simulink model "my_pv_system_3_ss_controller"  (Simulink 8.4)
settings: Solver=ode3  StartTime=0.0  StopTime=inf  FixedStep=5e-05  RelTol=1e-3
undefined symbols (not defined in the file or in its folder): another_event_name, my_event_name
libraries: powerlib_meascontrol x7, opal_lib x6, simulink x2, rtlab x1, powerlib x1
Description:
  | Model of a simple control system for use iin training.
settings Model: Creator=Paul Baracos  LastModifiedBy=jiang  BufferReuse=off
settings DataIOCC: SaveOutput=off  SaveTime=off  SignalLoggingName=sigsOut
settings OptimizationCC: BlockReduction=off  BooleanDataType=off  OptimizeBlockIOStorage=off  BufferReuse=off  GlobalBufferReuse=off  ExpressionFolding=off  ExpressionDepthLimit=128  LocalBlockOutputs=off  InitFltsAndDblsToZero=on
settings DebuggingCC: SaveWithParameterizedLinksMsg=none  SignalResolutionControl=TryResolveAllWithWarning  SolverPrmCheckMsg=none  MultiTaskDSMMsg=warning  MultiTaskCondExecSysMsg=none  StateNameClashWarn=none
settings HardwareCC: TargetHWDeviceType=32-bit Generic  TargetUnknown=on  ProdEqTarget=off
settings RTWCC: GenCodeOnly=on  IncludeERTFirstTime=on
settings GRTTargetCC: TargetFcnLib=ansi_tfl_tmw.mat
settings ConfigurationSet: Description=SimMechanics 2G

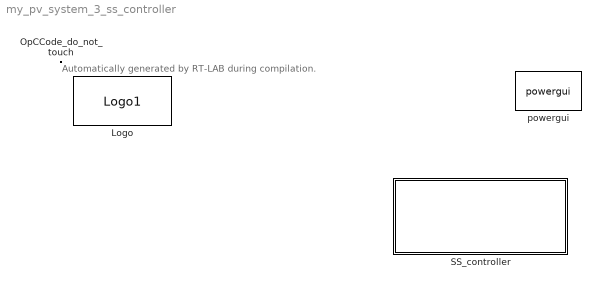
== system my_pv_system_3_ss_controller ==
  note: Automatically generated by RT-LAB during compilation.
  Logo : opal_lib/Logo1  vide=[]
  OpCCode_do_not_touch : opal_lib/Communication/OpCCode  SystemSampleTime=-1
  SS_controller : Subsystem
  powergui : powerlib/powergui  SimulationMode=Discrete  SolverType=Tustin/Backward Euler (TBE)  SampleTime=5e-05  frequency=60  SPID=off  DisableSnubberDevices=off  DisableRonSwitches=off  DisableVfSwitches=off  SwTol=0  DisplayEquations=off  Interpol=off  methode=off  Ts=100  frequencyindice=50  Pbase=100e6  ErrMax=1e-4  Iterations=50  UnitsV=kV  UnitsW=MW  FunctionMessages=off  echomessages=off  HookPort=off  EnableUseOfTLC=off  x0status=blocks  RestoreLinks=warning  ResistiveCurrentMeasurement=off  Frange=[0:2:500]  Ylog=off  Xlog=on  ShowGrid=off  save=off  variable=ZData  structure=0  ZoomFFT=off  StartTime=0.0  cycles=1  DisplayStyle=1  fundamental=60  FreqAxis=off  MaxFrequency=1000  frequencyindicesteady=1  RmsSteady=1  display=off

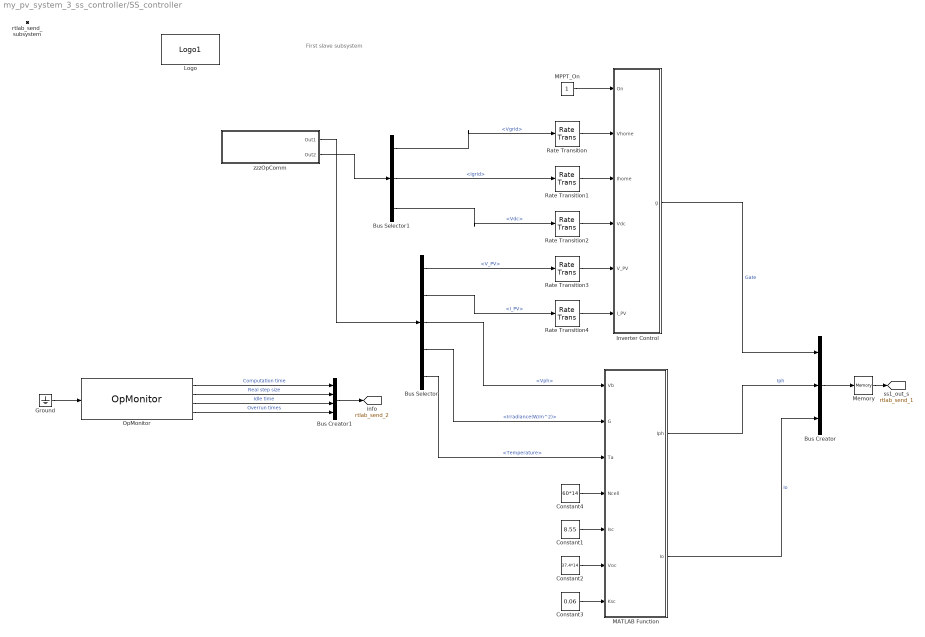
== system my_pv_system_3_ss_controller/SS_controller ==
  note: First slave subsystem
  Bus Creator : BusCreator  Inputs=3
  Bus Creator1 : BusCreator
  Bus Selector : BusSelector  OutputSignals=V_PV,I_PV,Vph,Irradiance(W/m^2),Temperature
  Bus Selector1 : BusSelector  OutputSignals=Vgrid,Igrid,Vdc
  Constant1 : Constant  Value=8.55
  Constant2 : Constant  Value=37.4*14
  Constant3 : Constant  Value=0.06
  Constant4 : Constant  Value=60*14
  Ground : Ground
  Inverter Control : Subsystem  mask(Inverter Control){Pnom=3500, Fnom=50, Vnom_prim=240, Vnom_dc=400, Increment_MPPT=0.003, Limits_MPPT=[ 450 375 ], Vdc_ref_Init=425, Kp_VDCreg=12, Ki_VDCreg=200, Kp_Ireg=0.15, Ki_Ireg=6.6, RLff=[ 0.002 0.20 ], Fc=4000, PWMmode12=Unipolar, Ts_Control=50e-6, Ts_PWMgenerator=50e-6}
      mask prompts: Pnom "Power (VA)"; Fnom "Frequency (Hz)"; Vnom_prim "Primary voltage (Vrms LL)"; Vnom_dc "DC voltage (V)"; Increment_MPPT "Output increment (V)"; Limits_MPPT "Output limits [ Upper  Lower ]"; Vdc_ref_Init "Output initial value (V)"; Kp_VDCreg "Proportional gain"; Ki_VDCreg "Integral gain"; Kp_Ireg "Proportional gain"; Ki_Ireg "Integral gain"; RLff "Feedforward Values [Rff Lff] (pu)"; Fc "Carrier frequency (Hz)"; PWMmode12 "PWM method"; Ts_Control "Control systems"; Ts_PWMgenerator "PWM generator"
      mask help:
      | The main components of the Inverter Control are:
      | 1. PLL & Measurements
      | 2. Maximum Power Point Tracker System (MPPT) using a Perturb & Observe algorithm
      | 3. DC Voltage Regulator
      | 4. Current Regulator
      | 5. PWM Modulator
      mask init:
      | blockName=gcb;
      | if PWMmode12==1
      |     set_param([blockName,'/','PWM_Generator'],'ModulatorType','Single-phase full-bridge (4 pulses)')
      | else
      |     set_param([blockName,'/','PWM_Generator'],'ModulatorType','Single-phase full-bridge - Bipolar modulation (4 pulses)')
      | end
      mask TypeOptions PWMmode12: Unipolar | Bipolar
  Logo : opal_lib/Logo1  vide=[]
  MATLAB Function : MATLAB Function  TreatAsAtomicUnit=on
  MPPT_On : Constant
  Memory : Memory  InheritSampleTime=on
  OpMonitor : rtlab/Monitoring/OpMonitor  compute_time=on  real_step=on  idle_time=on  nb_overruns=on  user_time=off  user_name=my_event_name,another_event_name
  Rate Transition{,1..4} (5 alike) : RateTransition
  rtlab_send_subsystem : Subsystem  Priority=-100
      mask Display: text(0,0,'');
  zzzOpComm : Subsystem
      mask init:
      | opmaskdisplay('maskdisplay_block',gcb,'disp(''OpComm'')');
      mask Display:
      | patch([0 0.5 0.7 0],[1 1 0 0],[0.7 0.75 0.9]);
      | patch([1 0.53 0.73 1],[1 1 0 0],[1 0.8 0.7]);
      | plot([0 0 1 1 0],[0 1 1 0 0]);
      | disp('OpComm')
  tag scope: rtlab_send_1=global, rtlab_send_2=global
  wires:
  Memory/1 -> [rtlab_send_1]
  MPPT_On/1 -> Inverter Control/1(On)
  Rate Transition/1 -> Inverter Control/2(Vhome)
  Rate Transition1/1 -> Inverter Control/3(Ihome)
  Rate Transition2/1 -> Inverter Control/4(Vdc)
  Rate Transition3/1 -> Inverter Control/5(V_PV)
  Rate Transition4/1 -> Inverter Control/6(I_PV)
  zzzOpComm/2(Out2) -> Bus Selector1/1
  Bus Selector1/1 -> Rate Transition/1  "<Vgrid>"
  Bus Selector1/2 -> Rate Transition1/1  "<Igrid>"
  Bus Selector1/3 -> Rate Transition2/1  "<Vdc>"
  zzzOpComm/1(Out1) -> Bus Selector/1
  Bus Selector/1 -> Rate Transition3/1  "<V_PV>"
  Bus Selector/2 -> Rate Transition4/1  "<I_PV>"
  Constant4/1 -> MATLAB Function/4(Ncell)
  Constant1/1 -> MATLAB Function/5(Isc)
  Constant2/1 -> MATLAB Function/6(Voc)
  Constant3/1 -> MATLAB Function/7(Ksc)
  Bus Creator/1 -> Memory/1
  Inverter Control/1(g) -> Bus Creator/1  "Gate"
  MATLAB Function/1(Iph) -> Bus Creator/2  "Iph"
  MATLAB Function/2(Io) -> Bus Creator/3  "Io"
  Bus Selector/3 -> MATLAB Function/1(Vb)  "<Vph>"
  Bus Selector/4 -> MATLAB Function/2(G)  "<Irradiance(W/m^2)>"
  Bus Selector/5 -> MATLAB Function/3(Ta)  "<Temperature>"
  Bus Creator1/1 -> [rtlab_send_2]
  OpMonitor/3 -> Bus Creator1/3  "Idle time"
  OpMonitor/1 -> Bus Creator1/1  "Computation time"
  OpMonitor/2 -> Bus Creator1/2  "Real step size"
  OpMonitor/4 -> Bus Creator1/4  "Overrun times"
  Ground/1 -> OpMonitor/1

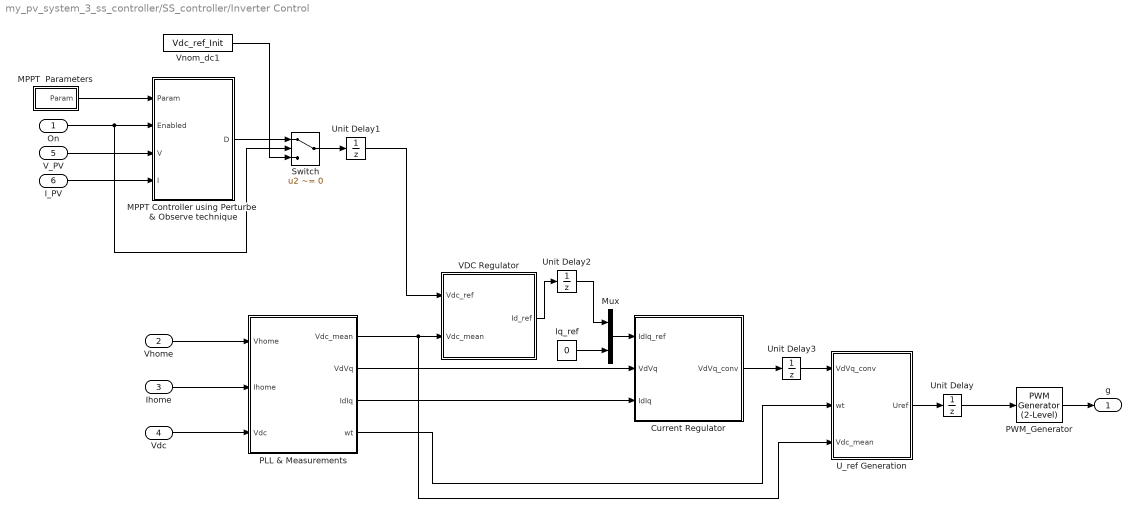
== system my_pv_system_3_ss_controller/SS_controller/Inverter Control ==
  On : Inport  PortDimensions=1
  Vhome : Inport  Port=2  PortDimensions=1
  Ihome : Inport  Port=3  PortDimensions=1
  Vdc : Inport  Port=4  PortDimensions=1
  V_PV : Inport  Port=5  PortDimensions=1
  I_PV : Inport  Port=6  PortDimensions=1
  Current Regulator : Subsystem
  Iq_ref : Constant  Value=0
  MPPT  Parameters : Subsystem
  "MPPT Controller using Perturbe  & Observe technique  " : MATLAB Function  TreatAsAtomicUnit=on
  Mux : Mux  Inputs=2
  PLL & Measurements : Subsystem
  PWM_Generator : powerlib_meascontrol/Pulse & Signal Generators/PWM Generator (2-Level)  ModulatorType=Single-phase full-bridge (4 pulses)  ModulatorMode=Unsynchronized  Fc=Fc  Pc=90  nF=27  MinMax="[ -1  1 ]"  SamplingTechnique=Natural  ModulatingSignals=off  m=0.8  Freq=60  Phase=0  Ts=Ts_PWMgenerator  ShowCarrierOutport=off
      settings: AttributesFormatString=%<ModulatorType>
  Switch : Switch  Criteria=u2 ~= 0
  "U_ref Generation " : Subsystem
  Unit Delay : UnitDelay  InitialCondition=0.1684  SampleTime=Ts_Control
  Unit Delay1 : UnitDelay  SampleTime=Ts_Control
  Unit Delay2 : UnitDelay  SampleTime=Ts_Control
  Unit Delay3 : UnitDelay  SampleTime=Ts_Control
  VDC Regulator : Subsystem
  Vnom_dc1 : Constant  Value=Vdc_ref_Init
  g : Outport
  wires:
  Iq_ref/1 -> Mux/2
  Vhome/1 -> PLL & Measurements/1(Vhome)
  Ihome/1 -> PLL & Measurements/2(Ihome)
  V_PV/1 -> "MPPT Controller using Perturbe  & Observe technique  "/3(V)
  I_PV/1 -> "MPPT Controller using Perturbe  & Observe technique  "/4(I)
  MPPT  Parameters/1(Param) -> "MPPT Controller using Perturbe  & Observe technique  "/1(Param)
  On/1 -> "MPPT Controller using Perturbe  & Observe technique  "/2(Enabled), Switch/2
  Unit Delay/1 -> PWM_Generator/1
  "MPPT Controller using Perturbe  & Observe technique  "/1(D) -> Switch/1
  Vdc/1 -> PLL & Measurements/3(Vdc)
  Vnom_dc1/1 -> Switch/3
  PLL & Measurements/2(VdVq) -> Current Regulator/2(VdVq)
  PLL & Measurements/3(IdIq) -> Current Regulator/3(IdIq)
  Mux/1 -> Current Regulator/1(IdIq_ref)
  PLL & Measurements/1(Vdc_mean) -> "U_ref Generation "/3(Vdc_mean), VDC Regulator/2(Vdc_mean)
  PLL & Measurements/4(wt) -> "U_ref Generation "/2(wt)
  "U_ref Generation "/1(Uref) -> Unit Delay/1
  PWM_Generator/1 -> g/1
  Switch/1 -> Unit Delay1/1
  Unit Delay1/1 -> VDC Regulator/1(Vdc_ref)
  VDC Regulator/1(Id_ref) -> Unit Delay2/1
  Unit Delay2/1 -> Mux/1
  Current Regulator/1(VdVq_conv) -> Unit Delay3/1
  Unit Delay3/1 -> "U_ref Generation "/1(VdVq_conv)

== system my_pv_system_3_ss_controller/SS_controller/rtlab_send_subsystem ==
  Subsystem2 : Subsystem
  Subsystem4 : Subsystem  Priority=-200000  TreatAsAtomicUnit=on
  wires:
  [rtlab_send_2] -> Subsystem2/1(In1)
  [rtlab_send_1] -> Subsystem4/1(In1)

== system my_pv_system_3_ss_controller/SS_controller/zzzOpComm ==
  Demux_1 : Demux  Outputs="[6  6]"
  Receive_1 : opal_lib/Communication/OpRec_rt  src=1  Data_width=12  st=5e-05
  busStruct : Subsystem
  Out1 : Outport
  Out2 : Outport  Port=2
  wires:
  Demux_1/2 -> busStruct/2(In2)
  Demux_1/1 -> busStruct/1(In1)
  busStruct/2(Out2) -> Out2/1
  busStruct/1(Out1) -> Out1/1
  Receive_1/1 -> Demux_1/1

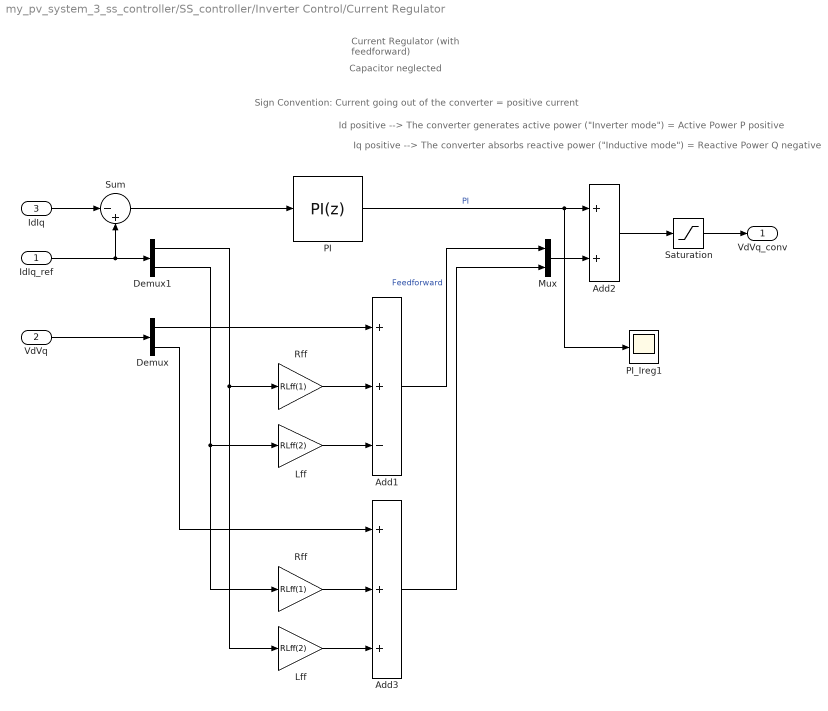
== system my_pv_system_3_ss_controller/SS_controller/Inverter Control/Current Regulator ==
  note: Id positive --> The converter generates active power ("Inverter mode") = Active Power P positive
  note: Iq positive --> The converter absorbs reactive power ("Inductive mode") = Reactive Power Q negative
  note: Sign Convention: Current going out of the converter = positive current
  note: Current Regulator
      | (with feedforward)
  note: Capacitor neglected
  IdIq_ref : Inport  PortDimensions=2
  VdVq : Inport  Port=2  PortDimensions=2
  IdIq : Inport  Port=3  PortDimensions=2
  Add1 : Sum  Inputs=++-
  Add2 : Sum
  Add3 : Sum  Inputs=+++
  Demux : Demux  Outputs=2
  Demux1 : Demux  Outputs=2
  Lff : Gain  Gain=RLff(2)  SaturateOnIntegerOverflow=on  OutDataTypeStr=Inherit: Same as input  ParamDataTypeStr=Inherit: Same as input
  "Lff  " : Gain  Gain=RLff(2)  SaturateOnIntegerOverflow=on  OutDataTypeStr=Inherit: Same as input  ParamDataTypeStr=Inherit: Same as input
  Mux : Mux  Inputs=2
  PI : simulink/Continuous/PID Controller  Controller=PI  TimeDomain=Discrete-time  SampleTime=Ts_Control  IntegratorMethod=Forward Euler  FilterMethod=Forward Euler  Form=Parallel  P=Kp_Ireg  I=Ki_Ireg  D=0  N=100  InitialConditionSource=internal  InitialConditionForIntegrator=0  InitialConditionForFilter=0  ExternalReset=none  LimitOutput=on  UpperSaturationLimit=1.5  LowerSaturationLimit=-1.5  LinearizeAsGain=off  AntiWindupMode=none  Kb=1  TrackingMode=off  Kt=1  PParamMin=[]  PParamMax=[]  IParamMin=[]  IParamMax=[]  DParamMin=[]  DParamMax=[]  NParamMin=[]  NParamMax=[]  KbParamMin=[]  KbParamMax=[]  KtParamMin=[]  KtParamMax=[]  POutMin=[]  POutMax=[]  IOutMin=[]  IOutMax=[]  DOutMin=[]  DOutMax=[]  NOutMin=[]  NOutMax=[]  KbOutMin=[]  KbOutMax=[]  KtOutMin=[]  KtOutMax=[]  IntegratorOutMin=[]  IntegratorOutMax=[]  FilterOutMin=[]  FilterOutMax=[]  SumOutMin=[]  SumOutMax=[]  SumI1OutMin=[]  SumI1OutMax=[]  SumI2OutMin=[]  SumI2OutMax=[]  SumI3OutMin=[]  SumI3OutMax=[]  SumDOutMin=[]  SumDOutMax=[]  SaturationOutMin=[]  SaturationOutMax=[]  IntegratorContinuousStateAttributes=''  IntegratorStateMustResolveToSignalObject=off  IntegratorRTWStateStorageClass=Auto  FilterContinuousStateAttributes=''  FilterStateMustResolveToSignalObject=off  FilterRTWStateStorageClass=Auto  DifferentiatorICPrevScaledInput=0  DifferentiatorOutMin=[]  DifferentiatorOutMax=[]  UseFilter=on
  PI_Ireg1 : Scope
      settings: YMin=-0.25  YMax=0.45
  Rff : Gain  Gain=RLff(1)  SaturateOnIntegerOverflow=on  OutDataTypeStr=Inherit: Same as input  ParamDataTypeStr=Inherit: Same as input
  "Rff " : Gain  Gain=RLff(1)  SaturateOnIntegerOverflow=on  OutDataTypeStr=Inherit: Same as input  ParamDataTypeStr=Inherit: Same as input
  Saturation : Saturate  UpperLimit=1.5  LowerLimit=-1.5
  Sum : Sum  Inputs=|-+
  VdVq_conv : Outport
  wires:
  Add3/1 -> Mux/2
  Demux/2 -> Add3/1
  Add1/1 -> Mux/1  "Feedforward"
  Lff/1 -> Add3/3
  Rff/1 -> Add3/2
  Demux1/2 -> Rff/1, "Lff  "/1
  "Lff  "/1 -> Add1/3
  Demux1/1 -> Lff/1, "Rff "/1
  "Rff "/1 -> Add1/2
  Demux/1 -> Add1/1
  VdVq/1 -> Demux/1
  Saturation/1 -> VdVq_conv/1
  Add2/1 -> Saturation/1
  IdIq/1 -> Sum/1
  IdIq_ref/1 -> Demux1/1, Sum/2
  Sum/1 -> PI/1
  PI/1 -> Add2/1, PI_Ireg1/1  "PI"
  Mux/1 -> Add2/2

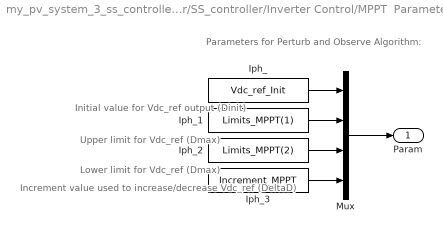
== system my_pv_system_3_ss_controller/SS_controller/Inverter Control/MPPT  Parameters ==
  note: Upper limit for Vdc_ref (Dmax)
  note: Increment value used to increase/decrease Vdc_ref (DeltaD)
  note: Initial value for Vdc_ref output (Dinit)
  note: Lower limit for Vdc_ref (Dmax)
  note: Parameters for Perturb and Observe Algorithm:
  Iph_ : Constant  Value=Vdc_ref_Init
  Iph_1 : Constant  Value=Limits_MPPT(1)
  Iph_2 : Constant  Value=Limits_MPPT(2)
  Iph_3 : Constant  Value=Increment_MPPT
  Mux : Mux
  Param : Outport
  wires:
  Iph_/1 -> Mux/1
  Iph_1/1 -> Mux/2
  Iph_2/1 -> Mux/3
  Iph_3/1 -> Mux/4
  Mux/1 -> Param/1

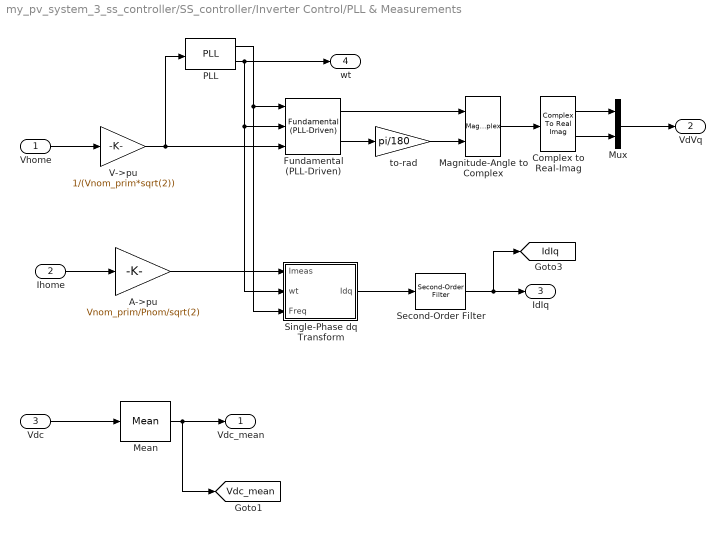
== system my_pv_system_3_ss_controller/SS_controller/Inverter Control/PLL & Measurements ==
  Vhome : Inport
  Ihome : Inport  Port=2
  Vdc : Inport  Port=3
  A->pu : Gain  Gain=Vnom_prim/Pnom/sqrt(2)  SaturateOnIntegerOverflow=on  OutDataTypeStr=Inherit: Same as input  ParamDataTypeStr=Inherit: Same as input
  Complex to Real-Imag : ComplexToRealImag
  Fundamental (PLL-Driven) : powerlib_meascontrol/Measurements/Fundamental (PLL-Driven)  Finit=Fnom  Fmin=45  InInit=[1, 0]  Ts=Ts_Control
  Magnitude-Angle to Complex : MagnitudeAngleToComplex
  Mean : powerlib_meascontrol/Measurements/Mean  Freq=Fnom  Vinit=Vdc_ref_Init  Ts=Ts_Control
  Mux : Mux  Inputs=2
  PLL : powerlib_meascontrol/PLL/PLL  Fmin=40  Par_Init=[0, Fnom]  ParK=[180, 3200, 1]  TcD=1e-4  MaxRateChangeFreq=12  FilterCutOffFreq=25  Ts=Ts_Control  AGC=on
  Second-Order Filter : powerlib_meascontrol/Filters/Second-Order Filter  FilterType=Lowpass  Fo=2000  Zeta=1  Ts=Ts_Control  Initialize=on  Vac_Init="[0,  0,  60;0,0,60]"  Vdc_Init=[0.9 0]  PlotResponse=off  FreqRange=[0, 500, 1]
  Single-Phase dq Transform : Subsystem
  V->pu : Gain  Gain=1/(Vnom_prim*sqrt(2))  SaturateOnIntegerOverflow=on  OutDataTypeStr=Inherit: Same as input  ParamDataTypeStr=Inherit: Same as input
  to-rad : Gain  Gain=pi/180
  Vdc_mean : Outport
  VdVq : Outport  Port=2
  IdIq : Outport  Port=3
  wt : Outport  Port=4
  tag scope: IdIq=global, Vdc_mean=global
  wires:
  Mean/1 -> Vdc_mean/1, [Vdc_mean]
  Vdc/1 -> Mean/1
  to-rad/1 -> Magnitude-Angle to Complex/2
  Mux/1 -> VdVq/1
  Complex to Real-Imag/2 -> Mux/2
  Complex to Real-Imag/1 -> Mux/1
  Magnitude-Angle to Complex/1 -> Complex to Real-Imag/1
  Fundamental (PLL-Driven)/2 -> to-rad/1
  Fundamental (PLL-Driven)/1 -> Magnitude-Angle to Complex/1
  A->pu/1 -> Single-Phase dq Transform/1(Imeas)
  PLL/1 -> Single-Phase dq Transform/3(Freq), Fundamental (PLL-Driven)/1
  PLL/2 -> wt/1, Fundamental (PLL-Driven)/2, Single-Phase dq Transform/2(wt)
  Ihome/1 -> A->pu/1
  Vhome/1 -> V->pu/1
  V->pu/1 -> Fundamental (PLL-Driven)/3, PLL/1
  Single-Phase dq Transform/1(Idq) -> Second-Order Filter/1
  Second-Order Filter/1 -> [IdIq], IdIq/1

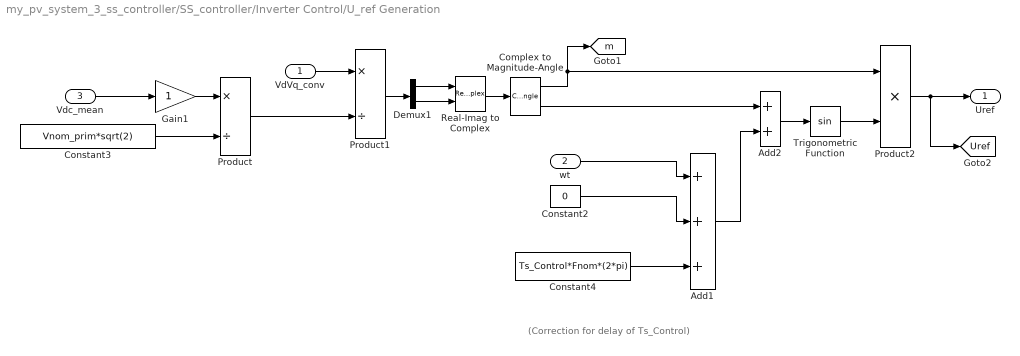
== system my_pv_system_3_ss_controller/SS_controller/Inverter Control/U_ref Generation  ==
  note: (Correction for delay of Ts_Control)
  VdVq_conv : Inport
  wt : Inport  Port=2
  Vdc_mean : Inport  Port=3
  Add1 : Sum  Inputs=+++
  Add2 : Sum
  Complex to Magnitude-Angle : ComplexToMagnitudeAngle
  Constant2 : Constant  Value=0
  Constant3 : Constant  Value=Vnom_prim*sqrt(2)
  Constant4 : Constant  Value=Ts_Control*Fnom*(2*pi)
  Demux1 : Demux  Outputs=2
  Gain1 : Gain
  Product : Product  Inputs=*/  RndMeth=Zero
  Product1 : Product  Inputs=*/  RndMeth=Zero
  Product2 : Product  Inputs=**  RndMeth=Zero
  Real-Imag to Complex : RealImagToComplex
  Trigonometric Function : Trigonometry
  Uref : Outport
  tag scope: Uref=global, m=global
  wires:
  VdVq_conv/1 -> Product1/1
  Product2/1 -> Uref/1, [Uref]
  Vdc_mean/1 -> Gain1/1
  Constant4/1 -> Add1/3
  wt/1 -> Add1/1
  Trigonometric Function/1 -> Product2/2
  Complex to Magnitude-Angle/1 -> [m], Product2/1
  Add2/1 -> Trigonometric Function/1
  Add1/1 -> Add2/2
  Complex to Magnitude-Angle/2 -> Add2/1
  Product/1 -> Product1/2
  Constant3/1 -> Product/2
  Constant2/1 -> Add1/2
  Demux1/2 -> Real-Imag to Complex/2
  Demux1/1 -> Real-Imag to Complex/1
  Real-Imag to Complex/1 -> Complex to Magnitude-Angle/1
  Gain1/1 -> Product/1
  Product1/1 -> Demux1/1

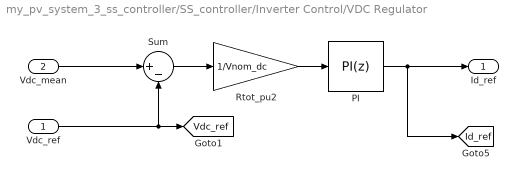
== system my_pv_system_3_ss_controller/SS_controller/Inverter Control/VDC Regulator ==
  Vdc_ref : Inport  PortDimensions=1
  Vdc_mean : Inport  Port=2  PortDimensions=1
  PI : simulink/Continuous/PID Controller  Controller=PI  TimeDomain=Discrete-time  SampleTime=Ts_Control  IntegratorMethod=Trapezoidal  FilterMethod=Forward Euler  Form=Parallel  P=Kp_VDCreg  I=Ki_VDCreg  D=0  N=100  InitialConditionSource=internal  InitialConditionForIntegrator=0.9226  InitialConditionForFilter=0  ExternalReset=none  LimitOutput=on  UpperSaturationLimit=1.5  LowerSaturationLimit=-1.5  LinearizeAsGain=off  AntiWindupMode=none  Kb=1  TrackingMode=off  Kt=1  PParamMin=[]  PParamMax=[]  IParamMin=[]  IParamMax=[]  DParamMin=[]  DParamMax=[]  NParamMin=[]  NParamMax=[]  KbParamMin=[]  KbParamMax=[]  KtParamMin=[]  KtParamMax=[]  POutMin=[]  POutMax=[]  IOutMin=[]  IOutMax=[]  DOutMin=[]  DOutMax=[]  NOutMin=[]  NOutMax=[]  KbOutMin=[]  KbOutMax=[]  KtOutMin=[]  KtOutMax=[]  IntegratorOutMin=[]  IntegratorOutMax=[]  FilterOutMin=[]  FilterOutMax=[]  SumOutMin=[]  SumOutMax=[]  SumI1OutMin=[]  SumI1OutMax=[]  SumI2OutMin=[]  SumI2OutMax=[]  SumI3OutMin=[]  SumI3OutMax=[]  SumDOutMin=[]  SumDOutMax=[]  SaturationOutMin=[]  SaturationOutMax=[]  IntegratorContinuousStateAttributes=''  IntegratorStateMustResolveToSignalObject=off  IntegratorRTWStateStorageClass=Auto  FilterContinuousStateAttributes=''  FilterStateMustResolveToSignalObject=off  FilterRTWStateStorageClass=Auto  DifferentiatorICPrevScaledInput=0  DifferentiatorOutMin=[]  DifferentiatorOutMax=[]  UseFilter=on
  Rtot_pu2 : Gain  Gain=1/Vnom_dc  SaturateOnIntegerOverflow=on  OutDataTypeStr=Inherit: Same as input  ParamDataTypeStr=Inherit: Same as input
  Sum : Sum  Inputs=|+-
  Id_ref : Outport  InitialOutput=0
  tag scope: Id_ref=global, Vdc_ref=global
  wires:
  Rtot_pu2/1 -> PI/1
  Vdc_ref/1 -> Sum/2, [Vdc_ref]
  Vdc_mean/1 -> Sum/1
  Sum/1 -> Rtot_pu2/1
  PI/1 -> Id_ref/1, [Id_ref]

== system my_pv_system_3_ss_controller/SS_controller/rtlab_send_subsystem/Subsystem2 ==
  In1 : Inport
  Mux : Mux  Inputs=1
  Send2 : opal_lib/Communication/OpSendToNT  Acqu_group=2
  wires:
  Mux/1 -> Send2/1
  In1/1 -> Mux/1

== system my_pv_system_3_ss_controller/SS_controller/rtlab_send_subsystem/Subsystem4 ==
  In1 : Inport
  Mux : Mux  Inputs=1
  Send4 : opal_lib/Communication/OpSend_rt  dest=1  priority2=0  st=5e-05
  wires:
  Mux/1 -> Send4/1
  In1/1 -> Mux/1

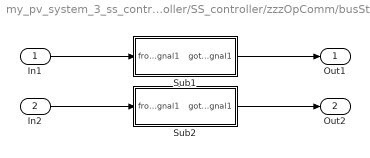
== system my_pv_system_3_ss_controller/SS_controller/zzzOpComm/busStruct ==
  In1 : Inport
  In2 : Inport  Port=2
  Sub1 : Subsystem
  Sub2 : Subsystem
  Out1 : Outport
  Out2 : Outport  Port=2
  wires:
  Sub2/1(goto_signal1) -> Out2/1
  In2/1 -> Sub2/1(from_signal1)
  Sub1/1(goto_signal1) -> Out1/1
  In1/1 -> Sub1/1(from_signal1)

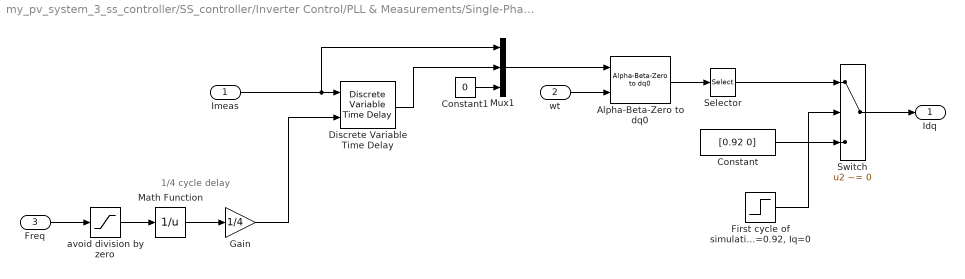
== system my_pv_system_3_ss_controller/SS_controller/Inverter Control/PLL & Measurements/Single-Phase dq Transform ==
  note: 1/4 cycle delay
  Imeas : Inport
  wt : Inport  Port=2
  Freq : Inport  Port=3
  Alpha-Beta-Zero to dq0 : powerlib_meascontrol/Transformations/Alpha-Beta-Zero to dq0  Alignment=90 degrees behind phase A axis
  Constant : Constant  Value=[0.92 0]
  Constant1 : Constant  Value=0
  Discrete Variable Time Delay : powerlib_meascontrol/Additional Components/Discrete Variable Time Delay  MaxDelay=1  InitialValue=0  Ts=Ts_Control  DFT=on
  "First cycle of simulation Id=0.92, Iq=0" : Step  Time=1/Fnom  SampleTime=Ts_Control
  Gain : Gain  Gain=1/4
  Math Function : Math  Operator=reciprocal  SaturateOnIntegerOverflow=on
  Mux1 : Mux  Inputs=3
  Selector : Selector  InputPortWidth=3  Indices=[1 2]
  Switch : Switch  Criteria=u2 ~= 0
  avoid division by zero : Saturate  UpperLimit=70  LowerLimit=40
  Idq : Outport
  wires:
  Constant1/1 -> Mux1/3
  Discrete Variable Time Delay/1 -> Mux1/2
  Mux1/1 -> Alpha-Beta-Zero to dq0/1
  Imeas/1 -> Discrete Variable Time Delay/1, Mux1/1
  wt/1 -> Alpha-Beta-Zero to dq0/2
  Alpha-Beta-Zero to dq0/1 -> Selector/1
  Freq/1 -> avoid division by zero/1
  avoid division by zero/1 -> Math Function/1
  Math Function/1 -> Gain/1
  Gain/1 -> Discrete Variable Time Delay/2
  Selector/1 -> Switch/1
  Switch/1 -> Idq/1
  Constant/1 -> Switch/3
  "First cycle of simulation Id=0.92, Iq=0"/1 -> Switch/2

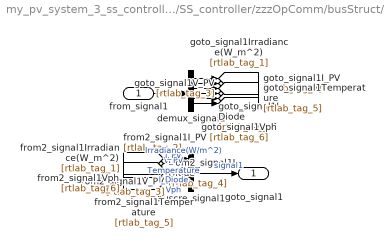
== system my_pv_system_3_ss_controller/SS_controller/zzzOpComm/busStruct/Sub1 ==
  from_signal1 : Inport
  buscre_signal1 : BusCreator  Inputs=6
  demux_signal1 : Demux  Outputs="[1  1  1  1  1  1]"
  goto_signal1 : Outport
  wires:
  buscre_signal1/1 -> goto_signal1/1  "signal1"
  [rtlab_tag_6] -> buscre_signal1/6  "Vph"
  [rtlab_tag_5] -> buscre_signal1/5  "Temperature"
  [rtlab_tag_4] -> buscre_signal1/4  "I_Diode"
  [rtlab_tag_3] -> buscre_signal1/3  "V_PV"
  [rtlab_tag_2] -> buscre_signal1/2  "I_PV"
  [rtlab_tag_1] -> buscre_signal1/1  "Irradiance(W/m^2)"
  demux_signal1/6 -> [rtlab_tag_6]
  demux_signal1/5 -> [rtlab_tag_5]
  demux_signal1/4 -> [rtlab_tag_4]
  demux_signal1/3 -> [rtlab_tag_3]
  demux_signal1/2 -> [rtlab_tag_2]
  demux_signal1/1 -> [rtlab_tag_1]
  from_signal1/1 -> demux_signal1/1

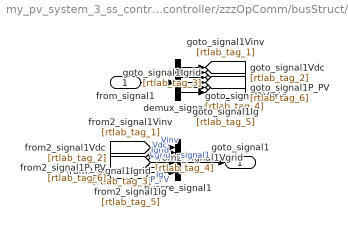
== system my_pv_system_3_ss_controller/SS_controller/zzzOpComm/busStruct/Sub2 ==
  from_signal1 : Inport
  buscre_signal1 : BusCreator  Inputs=6
  demux_signal1 : Demux  Outputs="[1  1  1  1  1  1]"
  goto_signal1 : Outport
  wires:
  buscre_signal1/1 -> goto_signal1/1  "signal1"
  [rtlab_tag_6] -> buscre_signal1/6  "P_PV"
  [rtlab_tag_5] -> buscre_signal1/5  "Ig"
  [rtlab_tag_4] -> buscre_signal1/4  "Vgrid"
  [rtlab_tag_3] -> buscre_signal1/3  "Igrid"
  [rtlab_tag_2] -> buscre_signal1/2  "Vdc"
  [rtlab_tag_1] -> buscre_signal1/1  "Vinv"
  demux_signal1/6 -> [rtlab_tag_6]
  demux_signal1/5 -> [rtlab_tag_5]
  demux_signal1/4 -> [rtlab_tag_4]
  demux_signal1/3 -> [rtlab_tag_3]
  demux_signal1/2 -> [rtlab_tag_2]
  demux_signal1/1 -> [rtlab_tag_1]
  from_signal1/1 -> demux_signal1/1

== matlab function SS_controller/MATLAB Function ==
  data: Vb input double; Iph output double; G input double; Ta input double; Ncell input double; Isc input double; Voc input double; Ksc input double; Io output double
function [Iph, Io] = PVpanel_new(Vb, G, Ta, Ncell, Isc, Voc, Ksc)

    toKelvin = 273;
    Ksc = Ksc / 100;
    G_ref = 1000;
    Ta_ref = 25 + toKelvin;
    Ta = Ta + toKelvin;
    deltaT = Ta - Ta_ref;
    k = 1.381e-23;
    q = 1.6e-19;
    eg = 1.12;                  % bandgap energy(1.12 eV)
    A = 1.3;                    % ideal factor
    a = Ncell * k * A * Ta / q;
    a_ref = Ncell * k * A * Ta_ref / q;
    Iph_ref = Isc;
    Voc_ref = Voc;
    Iph = G / G_ref * Iph_ref * (1 + Ksc * deltaT);
    Io_ref = Iph_ref / (exp(Voc_ref / a_ref) - 1);
    Io = Io_ref * (Ta / Ta_ref)^3 * ...
        exp((q * eg / A / k) * (1/Ta_ref - 1/Ta));
    Io = Io * (exp(Vb / a) - 1);

end

== matlab function SS_controller/Inverter Control/MPPT Controller using Perturbe & Observe technique  ==
  settings: updateMethod=DISCRETE  sampleTime=Ts_Control
  data: Param input double; Enabled input double; V input double; I input double; D output double
function D  = PandO(Param, Enabled, V, I)

% MPPT controller based on the Perturb & Observe algorithm.

% D output = Reference for DC link voltage (Vdc_ref) 
%
% Enabled input = 1 to enable the MPPT controller
% V input = PV array terminal voltage (V)
% I input = PV array current (A)
%
% Param input:
Dinit = Param(1);  %Initial value for Vdc_ref
Dmax = Param(2);   %Maximum value for Vdc_ref
Dmin = Param(3);   %Minimum value for Vdc_ref
deltaD = Param(4); %Increment value used to increase/decrease Vdc_ref
%  

persistent Vold Pold Dold;

dataType = 'double';

if isempty(Vold)
    Vold=0;
    Pold=0;
    Dold=Dinit;
end
P= V*I;
dV= V - Vold;
dP= P - Pold;

if dP ~= 0 & Enabled ~=0
    if dP < 0
        if dV < 0
            D = Dold + deltaD;
        else
            D = Dold - deltaD;
        end
    else
        if dV < 0
            D = Dold - deltaD;
        else
            D = Dold + deltaD;
        end    
    end
else D=Dold;
end

if D >= Dmax | D<= Dmin
    D=Dold;
end

Dold=D;
Vold=V;
Pold=P;
